simulink model "CuartoSuspension_simulink"  (R2023b)
settings: Solver=VariableStepAuto  StartTime=0.0  StopTime=10.0  RelTol=1e-3
values from neighbouring files (symbols this model uses):
  b1 = 1000    [CuartoSuspension.m]    (also in variablespractica3.m)
  f = 0    [CuartoSuspension.m]    (also in variablespractica3.m)
  k1 = 16182    [CuartoSuspension.m]    (also in variablespractica3.m)
  k2 = 19000    [CuartoSuspension.m]    (also in variablespractica3.m)
  m1 = 290    [CuartoSuspension.m]    (also in Parametros_Practica1.m = 0.2; Practica2.m = 0.1; variablespractica3.m)
  m2 = 59    [CuartoSuspension.m]    (also in Parametros_Practica1.m = 0.1; Practica2.m = 0.1; variablespractica3.m)
settings Model: Creator=edgar  LastModifiedBy=USER
settings ModelReferenceCC: EnableRefExpFcnMdlSchedulingChecks=on

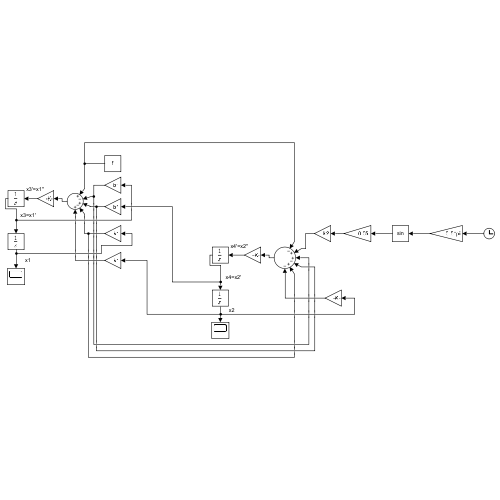
[thumbnail: Simulink's stored preview of the top-level diagram]
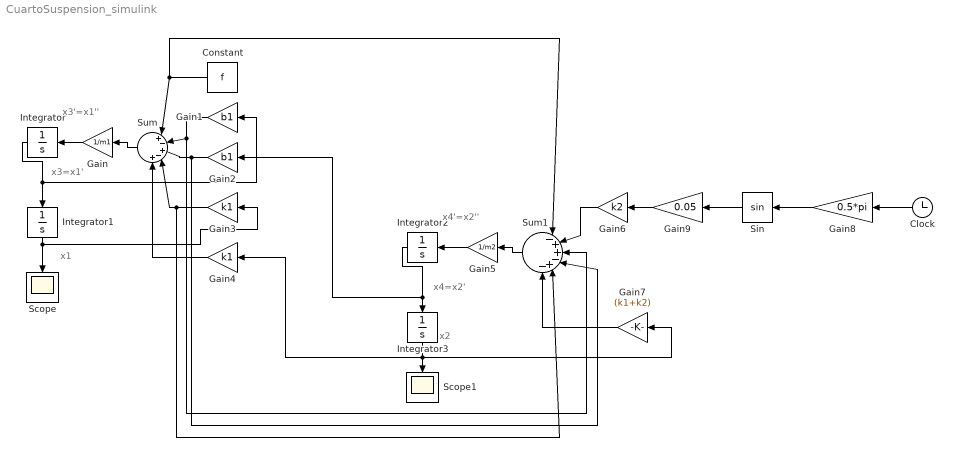
== system CuartoSuspension_simulink ==
  note: x3'=x1''
  note: x3=x1'
  note: x1
  note: x2
  note: x4'=x2''
  note: x4=x2'
  Clock : Clock
  Constant : Constant  Value=f
  Gain : Gain  Gain=1/m1
  Gain1 : Gain  Gain=b1
  Gain2 : Gain  Gain=b1
  Gain3 : Gain  Gain=k1
  Gain4 : Gain  Gain=k1
  Gain5 : Gain  Gain=1/m2
  Gain6 : Gain  Gain=k2
  Gain7 : Gain  Gain=(k1+k2)
  Gain8 : Gain  Gain=0.5*pi
  Gain9 : Gain  Gain=0.05
  Integrator{,1..3} (4 alike) : Integrator
  Scope : Scope
  Scope1 : Scope
  Sin : Trigonometry
  Sum : Sum  Inputs=|+-+-+
  Sum1 : Sum  Inputs=|-++-+-
  wires:
  Integrator/1 -> Gain1/1, Integrator1/1
  Integrator1/1 -> Gain3/1, Scope/1
  Gain/1 -> Integrator/1
  Sum/1 -> Gain/1
  Constant/1 -> Sum/1, Sum1/1
  Gain1/1 -> Sum1/3, Sum/2
  Gain2/1 -> Sum/3, Sum1/4
  Integrator3/1 -> Gain4/1, Scope1/1, Gain7/1
  Integrator2/1 -> Gain2/1, Integrator3/1
  Gain3/1 -> Sum1/5, Sum/4
  Gain4/1 -> Sum/5
  Gain5/1 -> Integrator2/1
  Sum1/1 -> Gain5/1
  Gain6/1 -> Sum1/2
  Gain7/1 -> Sum1/6
  Clock/1 -> Gain8/1
  Gain8/1 -> Sin/1
  Sin/1 -> Gain9/1
  Gain9/1 -> Gain6/1
